simulink model "dynamic_kinematic"  (R2021a)
settings: Solver=VariableStepAuto  StartTime=0.0  StopTime=10  RelTol=1e-3
libraries: pid_lib x2, robotmobilelib x1, fuzblock x1, simulink x1
settings Model: Creator=THANH DAT  LastModifiedBy=Admin

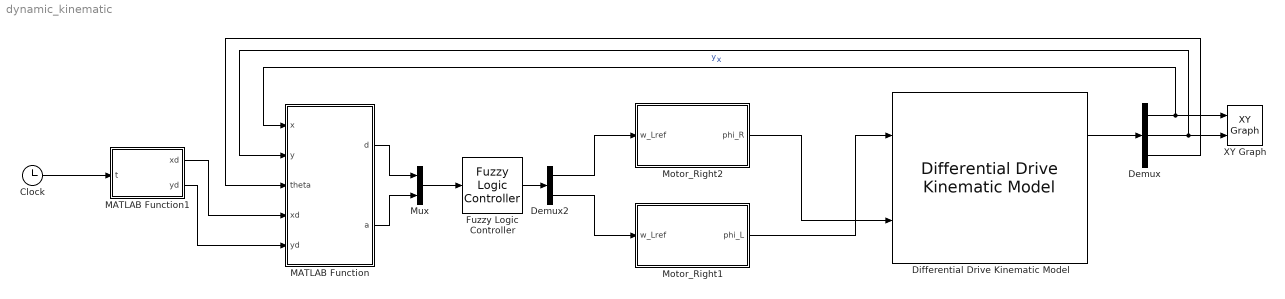
== system dynamic_kinematic ==
  Clock : Clock
  Demux : Demux  Outputs=3
  Demux2 : Demux  Outputs=2
  Differential Drive Kinematic Model : robotmobilelib/Differential Drive Kinematic Model  VehicleInputs=Wheel Speeds  WheelRadius=0.04  WheelSpeedRange=[-inf inf]  TrackWidth=0.2  InitialState=[0; 0; 0]  SimulateUsing=Interpreted execution
      settings: SourceProductBaseCode=RO
  Fuzzy Logic Controller : fuzblock/Fuzzy Logic  Controller  FIS='bangfuzzy.fis'  OutputSampleNumber=101  DataType=double  FuzzifiedInputs=off  RuleFiringStrengths=off  RuleOutputs=off  AggregatedOutputs=off  SimulateUsing=Interpreted execution  OutOfRangeInputValueMessage=warning  NoRuleFiredMessage=warning  EmptyOutputFuzzySetMessage=warning
  MATLAB Function : MATLAB Function  TreatAsAtomicUnit=on
  MATLAB Function1 : MATLAB Function  TreatAsAtomicUnit=on
  Motor_Right1 : Subsystem
  Motor_Right2 : Subsystem
  Mux : Mux  Inputs=2
  XY Graph : simulink/Sinks/XY Graph  xmin=-2  xmax=10  ymin=-2  ymax=2  st=-1
  wires:
  Differential Drive Kinematic Model/1 -> Demux/1
  Demux/1 -> MATLAB Function/1(x), XY Graph/1  "x"
  Demux/2 -> MATLAB Function/2(y), XY Graph/2  "y"
  Fuzzy Logic Controller/1 -> Demux2/1
  Mux/1 -> Fuzzy Logic Controller/1
  MATLAB Function/1(d) -> Mux/1
  MATLAB Function/2(a) -> Mux/2
  Demux/3 -> MATLAB Function/3(theta)
  MATLAB Function1/1(xd) -> MATLAB Function/4(xd)
  MATLAB Function1/2(yd) -> MATLAB Function/5(yd)
  Motor_Right2/1(phi_R) -> Differential Drive Kinematic Model/2
  Motor_Right1/1(phi_L) -> Differential Drive Kinematic Model/1
  Clock/1 -> MATLAB Function1/1(t)
  Demux2/1 -> Motor_Right2/1(w_Lref)
  Demux2/2 -> Motor_Right1/1(w_Lref)

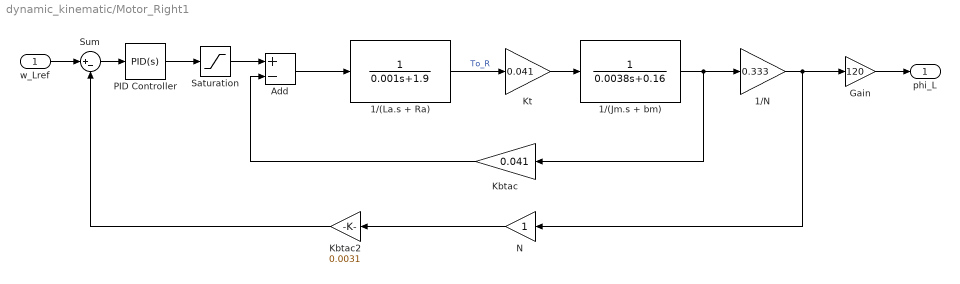
== system dynamic_kinematic/Motor_Right1 ==
  w_Lref : Inport
  1/(Jm.s + bm) : TransferFcn  Denominator=[0.0038 0.16]
  1/(La.s + Ra) : TransferFcn  Denominator=[0.001 1.9]
  1/N : Gain  Gain=0.333
  Add : Sum  Inputs=+-
  Gain : Gain  Gain=120
  Kbtac : Gain  Gain=0.041
  Kbtac2 : Gain  Gain=0.0031
  Kt : Gain  Gain=0.041
  N : Gain
  PID Controller : pid_lib/PID Controller  Controller=PID  Form=Parallel  TimeDomain=Continuous-time  UseExternalTs=off  SampleTime=-1  IntegratorMethod=Forward Euler  FilterMethod=Forward Euler  ControllerParametersSource=internal  P=1.2  I=1  D=0  UseFilter=on  N=100  TunerSelectOption=Transfer Function Based (PID Tuner App)  InitialConditionSource=internal  InitialConditionForIntegrator=0  InitialConditionForFilter=0  DifferentiatorICPrevScaledInput=0  ExternalReset=none  TrackingMode=off  Kt=1  LimitOutput=off  SatLimitsSource=internal  UpperSaturationLimit=inf  LowerSaturationLimit=-inf  LinearizeAsGain=on  AntiWindupMode=none  Kb=1  POutMin=[]  POutMax=[]  IOutMin=[]  IOutMax=[]  DOutMin=[]  DOutMax=[]  NOutMin=[]  NOutMax=[]  SumOutMin=[]  SumOutMax=[]  SaturationOutMin=[]  SaturationOutMax=[]  PParamMin=[]  PParamMax=[]  IParamMin=[]  IParamMax=[]  DParamMin=[]  DParamMax=[]  NParamMin=[]  NParamMax=[]  KbParamMin=[]  KbParamMax=[]  KtParamMin=[]  KtParamMax=[]  KbOutMin=[]  KbOutMax=[]  KtOutMin=[]  KtOutMax=[]  IntegratorOutMin=[]  IntegratorOutMax=[]  FilterOutMin=[]  FilterOutMax=[]  SumI1OutMin=[]  SumI1OutMax=[]  SumI2OutMin=[]  SumI2OutMax=[]  SumI3OutMin=[]  SumI3OutMax=[]  SumI4OutMin=[]  SumI4OutMax=[]  SumDOutMin=[]  SumDOutMax=[]  DifferentiatorOutMin=[]  DifferentiatorOutMax=[]  FilterDiffOutCoefMin=[]  FilterDiffOutCoefMax=[]  ReciprocalOutMin=[]  ReciprocalOutMax=[]  SumDenOutMin=[]  SumDenOutMax=[]  SumNumOutMin=[]  SumNumOutMax=[]  DivideOutMin=[]  DivideOutMax=[]  UdiffTsProdOutMin=[]  UdiffTsProdOutMax=[]  NTsProdOutMin=[]  NTsProdOutMax=[]  UintegralTsProdOutMin=[]  UintegralTsProdOutMax=[]  UngainTsProdOutMin=[]  UngainTsProdOutMax=[]  IntegratorContinuousStateAttributes=''  IntegratorStateMustResolveToSignalObject=off  IntegratorRTWStateStorageClass=Auto  FilterContinuousStateAttributes=''  FilterStateMustResolveToSignalObject=off  FilterRTWStateStorageClass=Auto  ParallelPVariant=InternalParameters  IdealPVariant=Disabled  IVariant=InternalParameters  DVariant=InternalParameters  IntegratorVariant=Continuous  SatVariant=Disabled  AWVariant=Passthrough  PCopyVariant=Disabled  TRVariant=Disabled  FdbkBlocksVariant=Forward  IdealPFdbkVariant=Disabled  SatFdbkVariant=Disabled  DerivativeFilterVariant=ContFilter  NVariant=InternalParameters  NCopyVariant=Disabled  FilterICVariant=InternalICsFilter  IntegratorICVariant=InternalICs  ExternalResetVariant=Disabled  TRSumVariant=Passthrough  SumFdbkVariant=Disabled  SumVariant=Sum_PID  TsampFilterVariant=InternalTs  TsampNgainVariant=Passthrough  TsampIntegralVariant=Passthrough  ExternalSaturationOutDataTypeStr=Inherit: Same as second input
  Saturation : Saturate  UpperLimit=12  LowerLimit=-12
  Sum : Sum  Inputs=|+-
  phi_L : Outport
  wires:
  Add/1 -> 1/(La.s + Ra)/1
  PID Controller/1 -> Saturation/1
  Saturation/1 -> Add/1
  Kt/1 -> 1/(Jm.s + bm)/1
  1/(La.s + Ra)/1 -> Kt/1  "To_R"
  1/(Jm.s + bm)/1 -> Kbtac/1, 1/N/1
  Kbtac2/1 -> Sum/2
  w_Lref/1 -> Sum/1
  Kbtac/1 -> Add/2
  Sum/1 -> PID Controller/1
  N/1 -> Kbtac2/1
  1/N/1 -> Gain/1, N/1
  Gain/1 -> phi_L/1

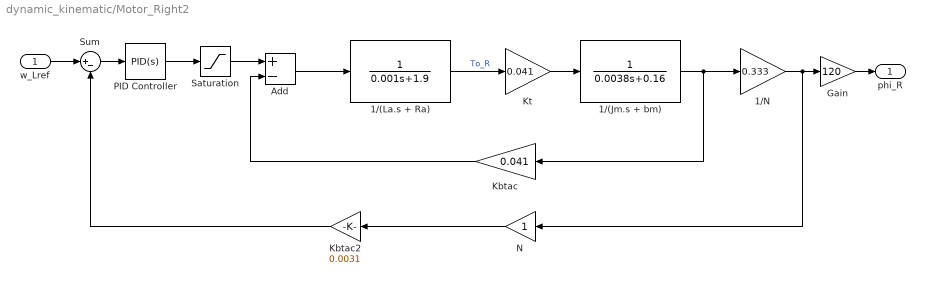
== system dynamic_kinematic/Motor_Right2 ==
  w_Lref : Inport
  1/(Jm.s + bm) : TransferFcn  Denominator=[0.0038 0.16]
  1/(La.s + Ra) : TransferFcn  Denominator=[0.001 1.9]
  1/N : Gain  Gain=0.333
  Add : Sum  Inputs=+-
  Gain : Gain  Gain=120
  Kbtac : Gain  Gain=0.041
  Kbtac2 : Gain  Gain=0.0031
  Kt : Gain  Gain=0.041
  N : Gain
  PID Controller : pid_lib/PID Controller  Controller=PID  Form=Parallel  TimeDomain=Continuous-time  UseExternalTs=off  SampleTime=-1  IntegratorMethod=Forward Euler  FilterMethod=Forward Euler  ControllerParametersSource=internal  P=1.2  I=1  D=0  UseFilter=on  N=100  TunerSelectOption=Transfer Function Based (PID Tuner App)  InitialConditionSource=internal  InitialConditionForIntegrator=0  InitialConditionForFilter=0  DifferentiatorICPrevScaledInput=0  ExternalReset=none  TrackingMode=off  Kt=1  LimitOutput=off  SatLimitsSource=internal  UpperSaturationLimit=inf  LowerSaturationLimit=-inf  LinearizeAsGain=on  AntiWindupMode=none  Kb=1  POutMin=[]  POutMax=[]  IOutMin=[]  IOutMax=[]  DOutMin=[]  DOutMax=[]  NOutMin=[]  NOutMax=[]  SumOutMin=[]  SumOutMax=[]  SaturationOutMin=[]  SaturationOutMax=[]  PParamMin=[]  PParamMax=[]  IParamMin=[]  IParamMax=[]  DParamMin=[]  DParamMax=[]  NParamMin=[]  NParamMax=[]  KbParamMin=[]  KbParamMax=[]  KtParamMin=[]  KtParamMax=[]  KbOutMin=[]  KbOutMax=[]  KtOutMin=[]  KtOutMax=[]  IntegratorOutMin=[]  IntegratorOutMax=[]  FilterOutMin=[]  FilterOutMax=[]  SumI1OutMin=[]  SumI1OutMax=[]  SumI2OutMin=[]  SumI2OutMax=[]  SumI3OutMin=[]  SumI3OutMax=[]  SumI4OutMin=[]  SumI4OutMax=[]  SumDOutMin=[]  SumDOutMax=[]  DifferentiatorOutMin=[]  DifferentiatorOutMax=[]  FilterDiffOutCoefMin=[]  FilterDiffOutCoefMax=[]  ReciprocalOutMin=[]  ReciprocalOutMax=[]  SumDenOutMin=[]  SumDenOutMax=[]  SumNumOutMin=[]  SumNumOutMax=[]  DivideOutMin=[]  DivideOutMax=[]  UdiffTsProdOutMin=[]  UdiffTsProdOutMax=[]  NTsProdOutMin=[]  NTsProdOutMax=[]  UintegralTsProdOutMin=[]  UintegralTsProdOutMax=[]  UngainTsProdOutMin=[]  UngainTsProdOutMax=[]  IntegratorContinuousStateAttributes=''  IntegratorStateMustResolveToSignalObject=off  IntegratorRTWStateStorageClass=Auto  FilterContinuousStateAttributes=''  FilterStateMustResolveToSignalObject=off  FilterRTWStateStorageClass=Auto  ParallelPVariant=InternalParameters  IdealPVariant=Disabled  IVariant=InternalParameters  DVariant=InternalParameters  IntegratorVariant=Continuous  SatVariant=Disabled  AWVariant=Passthrough  PCopyVariant=Disabled  TRVariant=Disabled  FdbkBlocksVariant=Forward  IdealPFdbkVariant=Disabled  SatFdbkVariant=Disabled  DerivativeFilterVariant=ContFilter  NVariant=InternalParameters  NCopyVariant=Disabled  FilterICVariant=InternalICsFilter  IntegratorICVariant=InternalICs  ExternalResetVariant=Disabled  TRSumVariant=Passthrough  SumFdbkVariant=Disabled  SumVariant=Sum_PID  TsampFilterVariant=InternalTs  TsampNgainVariant=Passthrough  TsampIntegralVariant=Passthrough  ExternalSaturationOutDataTypeStr=Inherit: Same as second input
  Saturation : Saturate  UpperLimit=12  LowerLimit=-12
  Sum : Sum  Inputs=|+-
  phi_R : Outport
  wires:
  Add/1 -> 1/(La.s + Ra)/1
  PID Controller/1 -> Saturation/1
  Saturation/1 -> Add/1
  Kt/1 -> 1/(Jm.s + bm)/1
  1/(La.s + Ra)/1 -> Kt/1  "To_R"
  1/(Jm.s + bm)/1 -> Kbtac/1, 1/N/1
  Kbtac2/1 -> Sum/2
  w_Lref/1 -> Sum/1
  Kbtac/1 -> Add/2
  Sum/1 -> PID Controller/1
  N/1 -> Kbtac2/1
  1/N/1 -> Gain/1, N/1
  Gain/1 -> phi_R/1

== matlab function dynamic_kinematic/MATLAB Function1 ==
  data: t input; xd output; yd output
function [xd,yd] = fcn(t)

xd = t;
yd = cos(t);

== matlab function dynamic_kinematic/MATLAB Function ==
  data: x input; d output; y input; theta input; xd input; yd input; a output
function [d,a] = boxuly(x,y,theta,xd,yd)

dx = xd-x;
dy = yd-y;
d=sqrt(dx^2+dy^2)-0.01;
thetad = atan2(dy,dx);
if (thetad-pi<theta)&&(theta<pi)&&(0<thetad)&&(thetad<pi)
a=thetad-theta;
elseif (-pi<theta)&&(theta<thetad-pi)&&(0<thetad)&&(thetad<pi)
a=thetad-theta-2*pi;
elseif (-pi<theta)&&(theta<pi-abs(thetad))&&(-pi<thetad)&&(thetad<0)
a=thetad-theta;
elseif (pi-abs(thetad)<theta)&&(theta<pi)&&(-pi<thetad)&&(thetad<0)
a=2*pi-(theta+abs(thetad));
else
    a=0;
end
